simulink model "Assignment1"  (R2014a)
settings: Solver=FixedStepDiscrete  StartTime=0.0  StopTime=2000  FixedStep=1  RelTol=1e-3
libraries: simulink x2, hdlsllib x2
settings Model: Creator=vu.du  LastModifiedBy=vu.du

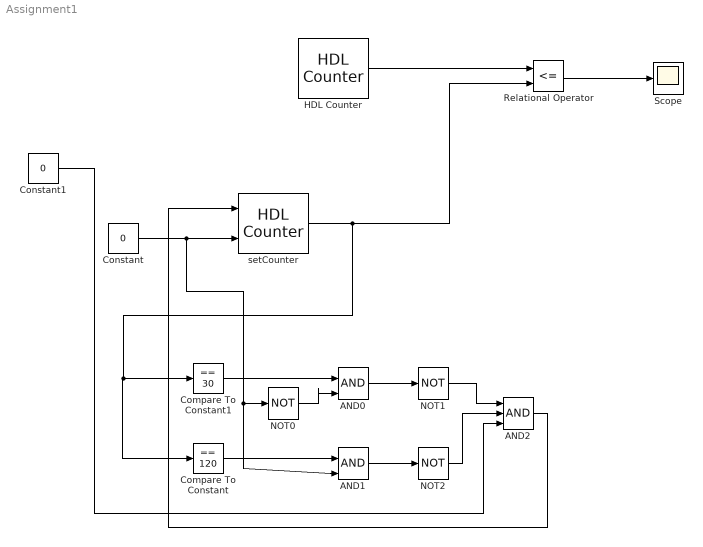
== system Assignment1 ==
  AND0 : Logic  IconShape=distinctive  AllPortsSameDT=off  OutDataTypeStr=boolean
  AND1 : Logic  IconShape=distinctive  AllPortsSameDT=off  OutDataTypeStr=boolean
  AND2 : Logic  Inputs=3  IconShape=distinctive  AllPortsSameDT=off  OutDataTypeStr=boolean
  Compare To Constant : simulink/Logic and Bit Operations/Compare To Constant  relop===  const=120  OutDataTypeStr=boolean
  Compare To Constant1 : simulink/Logic and Bit Operations/Compare To Constant  relop===  const=30  OutDataTypeStr=boolean
  Constant : Constant  Value=0  OutDataTypeStr=boolean
  Constant1 : Constant  Value=0  OutDataTypeStr=boolean
  HDL Counter : hdlsllib/HDL Operations/HDL Counter  CountType=Count limited  CountInit=0  CountStep=1  CountMax=1000  CountFromType=Initial value  CountFrom=0  CountResetPort=off  CountLoadPort=off  CountEnbPort=off  CountDirPort=off  CountDataType=Unsigned  CountWordLen=32  CountFracLen=0  CountSampTime=1
  NOT0 : Logic  Operator=NOT  IconShape=distinctive  AllPortsSameDT=off  OutDataTypeStr=boolean
  NOT1 : Logic  Operator=NOT  IconShape=distinctive  AllPortsSameDT=off  OutDataTypeStr=boolean
  NOT2 : Logic  Operator=NOT  IconShape=distinctive  AllPortsSameDT=off  OutDataTypeStr=boolean
  Relational Operator : RelationalOperator  Operator=<=  OutDataTypeStr=boolean
  Scope : Scope
  setCounter : hdlsllib/HDL Operations/HDL Counter  CountType=Count limited  CountInit=75  CountStep=6  CountMax=120  CountFromType=Specify  CountFrom=30  CountResetPort=off  CountLoadPort=off  CountEnbPort=on  CountDirPort=on  CountDataType=Unsigned  CountWordLen=32  CountFracLen=0  CountSampTime=1
  wires:
  setCounter/1 -> Compare To Constant/1, Compare To Constant1/1, Relational Operator/2
  HDL Counter/1 -> Relational Operator/1
  Constant/1 -> AND1/2, NOT0/1, setCounter/2
  Relational Operator/1 -> Scope/1
  Compare To Constant1/1 -> AND0/1
  NOT0/1 -> AND0/2
  Compare To Constant/1 -> AND1/1
  AND0/1 -> NOT1/1
  AND1/1 -> NOT2/1
  NOT1/1 -> AND2/1
  NOT2/1 -> AND2/2
  Constant1/1 -> AND2/3
  AND2/1 -> setCounter/1
